simulink model "sat_model_delivery"  (R2023b)
settings: Solver=ode5  StartTime=0.0  StopTime=2*T  RelTol=1e-3
undefined symbols (not defined in the file): a, alpha1, alpha12, alpha2, alpha22, alpha3, bias_earth, bias_mag, bias_sun, DiscIntNeverNeededParam, e, flag_h, FOV_earth, freq_acds, freq_act, freq_earth, freq_mag, freq_sun, gh, I_ext, I_retr, I_wheel, Iinv_ext, Iinv_retr, jb, k_gain, magnitude, max_dip, max_hdot, mu, n, noise_sd_mag, omega0, omegaE, rs, s0, s_h, s_m, s_s, tol, v_h, v_m, v_s, w_sat
libraries: simulink x16, vrlib x10, matrix_library x7, cstextras x4, cstblocks x1, simulink_extras x1
(part 1 of 3)
settings Model: Creator=danie  LastModifiedBy=danie

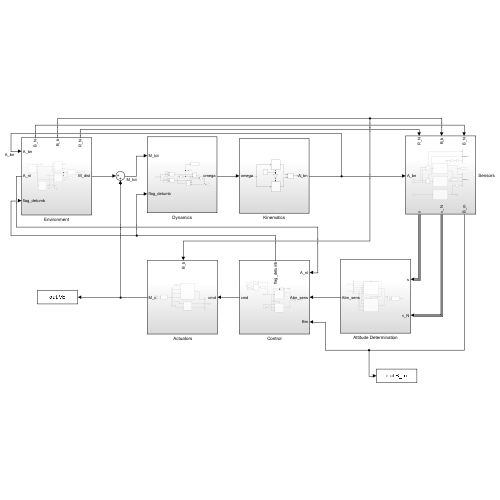
[thumbnail: Simulink's stored preview of the top-level diagram]
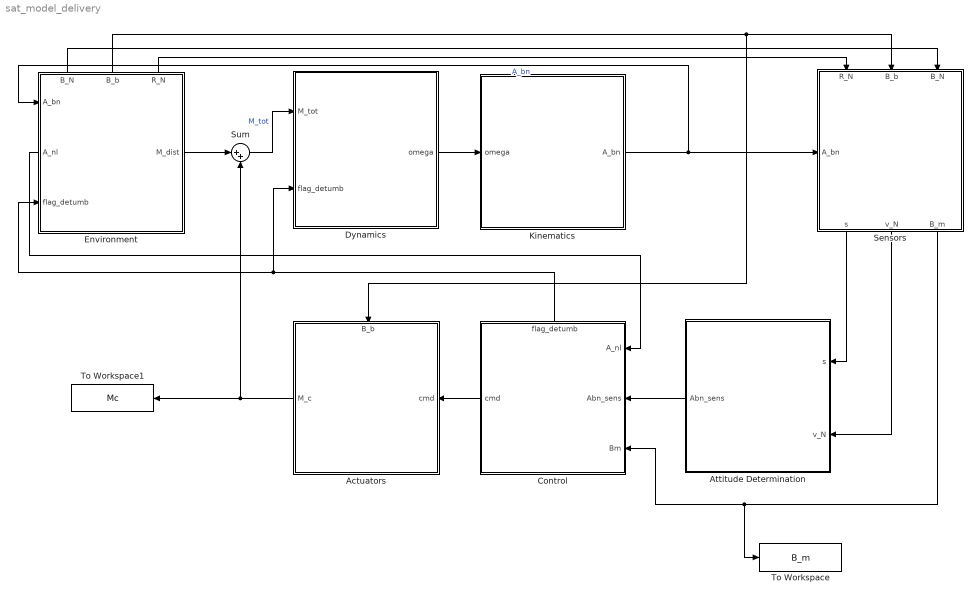
== system sat_model_delivery ==
  " Actuators" : Subsystem
      settings: PortSchema="{\"entries\":[{\"content\":{\"sides\":[{\"content\":{\"connectorIds\":[\"In1\"]},\"type\":\"ConnectorPlacement.EquallySpacedRectSide\",\"uuid\":\"5d6e642f-1157-4b0e-aa08-9ddf4ff16df7\"},{\"content\":{\"connectorIds\":[\"Out1\"],\"side\":\"RIGHT\"},\"type\":\"ConnectorPlacement.EquallySpacedRectSide\",\"uuid\":\"5847b5a1-e838-48cc-aba7-537ea27379c6\"},{\"content\":{\"connectorIds\":[\"In2\"],\"side\":\"TOP\"},\"type\":\"ConnectorPlacement.EquallySpacedRectSide\",\"uuid\":\"a1f0acea-f413-4d04-85a3-ab4e053335d5\"}]},\"type\":\"ConnectorPlacement.EquallySpacedConnector\",\"uuid\":\"33dffe5d-89c5-4628-a461-5573ab7b5256\"}],\"packageUris\":[\"http://schema.mathworks.com/mf0/Connector/R2020b\"],\"version\":\"1.0\"}"
  Attitude Determination : Subsystem
      settings: PortSchema="{\"entries\":[{\"content\":{\"sides\":[{\"content\":{\"connectorIds\":[\"Out1\"]},\"type\":\"ConnectorPlacement.EquallySpacedRectSide\",\"uuid\":\"730966cf-d0d7-44a0-92f0-b5324480e7cc\"},{\"content\":{\"connectorIds\":[\"In1\",\"In2\"],\"side\":\"RIGHT\"},\"type\":\"ConnectorPlacement.EquallySpacedRectSide\",\"uuid\":\"c83e6b57-46fe-4a45-9824-d3495e15bf6a\"},{\"content\":{\"side\":\"TOP\"},\"type\":\"ConnectorPlacement.EquallySpacedRectSide\",\"uuid\":\"4938c298-c2b3-45b7-bcb0-70b8132dabc6\"},{\"content\":{\"side\":\"BOTTOM\"},\"type\":\"ConnectorPlacement.EquallySpacedRectSide\",\"uuid\":\"6d6a244e-80db-423b-a0a5-9a5face48fcb\"}]},\"type\":\"ConnectorPlacement.EquallySpacedConnector\",\"uuid\":\"7eb6767d-3ff0-4577-86c9-ebc5e763f220\"}],\"packageUris\":[\"http://schema.mathworks.com/mf0/Connector/R2020b\"],\"version\":\"1.0\"}"
  Control : Subsystem
      settings: PortSchema="{\"entries\":[{\"content\":{\"sides\":[{\"content\":{\"connectorIds\":[\"In1\",\"In2\",\"In3\"]},\"type\":\"ConnectorPlacement.EquallySpacedRectSide\",\"uuid\":\"479db2a9-02dc-44e2-91e0-a22764ce85e5\"},{\"content\":{\"connectorIds\":[\"Out1\"],\"side\":\"RIGHT\"},\"type\":\"ConnectorPlacement.EquallySpacedRectSide\",\"uuid\":\"f4f8a6e1-932f-455d-9102-afbfd34f7a90\"},{\"content\":{\"connectorIds\":[\"Out2\"],\"side\":\"TOP\"},\"type\":\"ConnectorPlacement.EquallySpacedRectSide\",\"uuid\":\"6b9117e9-1db7-436f-b480-50cd5021b49c\"}]},\"type\":\"ConnectorPlacement.EquallySpacedConnector\",\"uuid\":\"5cd0260c-2101-4e31-9539-e0e89bfc4be8\"}],\"packageUris\":[\"http://schema.mathworks.com/mf0/Connector/R2020b\"],\"version\":\"1.0\"}"
  Dynamics : Subsystem
  Environment : Subsystem
      settings: PortSchema="{\"entries\":[{\"content\":{\"sides\":[{\"content\":{\"connectorIds\":[\"In1\",\"Out5\",\"In2\"]},\"type\":\"ConnectorPlacement.EquallySpacedRectSide\",\"uuid\":\"cd547eb7-7be0-4e5b-836c-c366b6478044\"},{\"content\":{\"connectorIds\":[\"Out1\"],\"side\":\"RIGHT\"},\"type\":\"ConnectorPlacement.EquallySpacedRectSide\",\"uuid\":\"e1dc659a-5264-4743-a04f-d64598214c88\"},{\"content\":{\"connectorIds\":[\"Out2\",\"Out3\",\"Out4\"],\"side\":\"TOP\"},\"type\":\"ConnectorPlacement.EquallySpacedRectSide\",\"uuid\":\"7e012610-9217-4888-a063-1dd5014a7789\"}]},\"type\":\"ConnectorPlacement.EquallySpacedConnector\",\"uuid\":\"403067f0-c93a-4211-8718-9c9152968794\"}],\"packageUris\":[\"http://schema.mathworks.com/mf0/Connector/R2020b\"],\"version\":\"1.0\"}"
  Kinematics : Subsystem
  Sensors : Subsystem
      settings: PortSchema="{\"entries\":[{\"content\":{\"sides\":[{\"content\":{\"connectorIds\":[\"In1\"]},\"type\":\"ConnectorPlacement.EquallySpacedRectSide\",\"uuid\":\"89361889-f7de-4872-ae0d-1858deeb7249\"},{\"content\":{\"side\":\"RIGHT\"},\"type\":\"ConnectorPlacement.EquallySpacedRectSide\",\"uuid\":\"dfd6afc4-03b7-4a72-bde7-03d61914b85e\"},{\"content\":{\"connectorIds\":[\"In2\",\"In3\",\"In4\"],\"side\":\"TOP\"},\"type\":\"ConnectorPlacement.EquallySpacedRectSide\",\"uuid\":\"ce9e53bd-32cb-428b-aff5-bfd70ec52f8d\"},{\"content\":{\"connectorIds\":[\"Out1\",\"Out2\",\"Out3\"],\"side\":\"BOTTOM\"},\"type\":\"ConnectorPlacement.EquallySpacedRectSide\",\"uuid\":\"2ad17a34-6232-44a6-b54d-45b43e2b5f52\"}]},\"type\":\"ConnectorPlacement.EquallySpacedConnector\",\"uuid\":\"a62cbf6d-d04c-4cf6-ac53-e5ea1ee04b12\"}],\"packageUris\":[\"http://schema.mathworks.com/mf0/Connector/R2020b\"],\"version\":\"1.0\"}"
  Sum : Sum  Inputs=|++
  To Workspace : ToWorkspace  VariableName=B_m  SampleTime=-1
  To Workspace1 : ToWorkspace  VariableName=Mc  SampleTime=-1
  wires:
  " Actuators"/1(M_c) -> To Workspace1/1, Sum/2
  Control/2(flag_detumb) -> Environment/2(flag_detumb), Dynamics/2(flag_detumb)
  Environment/2(B_N) -> Sensors/4(B_N)
  Control/1(cmd) -> " Actuators"/1(cmd)
  Environment/1(M_dist) -> Sum/1
  Kinematics/1(A_bn) -> Sensors/1(A_bn), Environment/1(A_bn)  "A_bn"
  Environment/4(R_N) -> Sensors/2(R_N)
  Attitude Determination/1(Abn_sens) -> Control/2(Abn_sens)
  Environment/3(B_b) -> " Actuators"/2(B_b), Sensors/3(B_b)
  Sensors/3(B_m) -> To Workspace/1, Control/3(Bm)
  Environment/5(A_nl) -> Control/1(A_nl)
  Sensors/1(s) -> Attitude Determination/1(s)
  Sensors/2(v_N) -> Attitude Determination/2(v_N)
  Dynamics/1(omega) -> Kinematics/1(omega)
  Sum/1 -> Dynamics/1(M_tot)  "M_tot"

== system sat_model_delivery/ Actuators ==
  cmd : Inport
  B_b : Inport  Port=2
  Constant : Constant  Value=5
  Demux : Demux  Outputs=5
  Discrete Varying Lowpass : Subsystem  mask(Discrete Varying Lowpass){N=2, w0=0, Ts=1/30}
      mask prompts: N "Control:simulink:VaryingLowpassLabel1"; w0 "Control:simulink:VaryingLowpassLabel2"; Ts "Control:simulink:VaryingLowpassLabel3"
      mask help: Control:simulink:VaryingLowpass2
      mask init:
      | if N~=round(N)
      |    hCB = get_param(gcb,'handle');
      |    DAStudio.slerror('Control:simulink:InvalidOrder',hCB)
      | elseif w0*Ts>=pi
      |    hCB = get_param(gcb,'handle');
      |    DAStudio.slerror('Control:simulink:InvalidPrewarp',hCB)
      | end
      | SimStatus = get_param(bdroot,'SimulationStatus');
      | if any(strcmp(SimStatus,{'initializing','updating','stopped'}))
      |    controllib.internal.blocks.varying.varyingLP(gcb,N,Ts)
      | end
      settings: LibrarySourceBlock=cstblocks/Linear Parameter Varying/Discrete Varying Lowpass
      mask Help: eval('helpview(''control'',''VaryingLowpassDT'');')
      mask DialogControl N Prompt: Filter order:
      mask DialogControl w0 Prompt: Pre-warping frequency w0 (rad/s):
      mask DialogControl Ts Prompt: Sample time Ts:
      mask Display:
      | image('lowpass_dt.png',[0.1 0 0.8 1]);
      | port_label('input', 2, 'freq');
  Magnetorquers : Subsystem
  Reaction wheels : Subsystem
  Sum : Sum  Inputs=+++
  M_c : Outport
  wires:
  Sum/1 -> M_c/1
  Constant/1 -> Discrete Varying Lowpass/2(frequency)
  Discrete Varying Lowpass/1(y) -> Demux/1
  cmd/1 -> Discrete Varying Lowpass/1(u)
  Demux/1 -> Magnetorquers/2(Dx)  "Dx"
  Demux/2 -> Magnetorquers/3(Dy)  "Dy"
  B_b/1 -> Magnetorquers/1(B_b)
  Demux/3 -> Magnetorquers/4(Dz)  "Dz"
  Magnetorquers/1(M_mag) -> Sum/1
  Demux/4 -> Reaction wheels/1(-h_dot_x)  "-h_dot_x"
  Demux/5 -> Reaction wheels/2(-h_dot_y)  "-h_dot_y"
  Reaction wheels/1(M_wheel_x) -> Sum/2
  Reaction wheels/2(M_wheel_y) -> Sum/3

== system sat_model_delivery/Attitude Determination ==
  s : Inport
  v_N : Inport  Port=2
  Bus Selector : BusSelector  OutputSignals=flag_h,s_h,s_s,s_m
  Bus Selector1 : BusSelector  OutputSignals=v_h,v_s,v_m
  Constant : Constant  Value=0.5
  Discrete Varying Lowpass : cstblocks/Linear Parameter Varying/Discrete Varying Lowpass  N=2  w0=0  Ts=1/freq_acds
  Merge : Merge
  NOT : Logic  Operator=NOT  IconShape=distinctive  AllPortsSameDT=off  OutDataTypeStr=boolean
  Three Sensors : Subsystem  TreatAsAtomicUnit=on
  Two Sensors : Subsystem  TreatAsAtomicUnit=on
  Abn_sens : Outport
  wires:
  Bus Selector/1 -> Three Sensors/Enable, NOT/1  "<flag_h>"
  NOT/1 -> Two Sensors/Enable
  Three Sensors/1(Abn_sens) -> Merge/1
  Two Sensors/1(A_bn_sens) -> Merge/2
  s/1 -> Bus Selector/1
  Bus Selector/2 -> Three Sensors/1(s1)  "<s_h>"
  Bus Selector/3 -> Two Sensors/1(s1), Three Sensors/2(s2)  "<s_s>"
  Bus Selector/4 -> Two Sensors/2(s2), Three Sensors/3(s3)  "<s_m>"
  v_N/1 -> Bus Selector1/1
  Bus Selector1/1 -> Three Sensors/4(v1)  "<v_h>"
  Bus Selector1/2 -> Two Sensors/3(v1), Three Sensors/5(v2)  "<v_s>"
  Bus Selector1/3 -> Two Sensors/4(v2), Three Sensors/6(v3)  "<v_m>"
  Merge/1 -> Discrete Varying Lowpass/1
  Discrete Varying Lowpass/1 -> Abn_sens/1
  Constant/1 -> Discrete Varying Lowpass/2

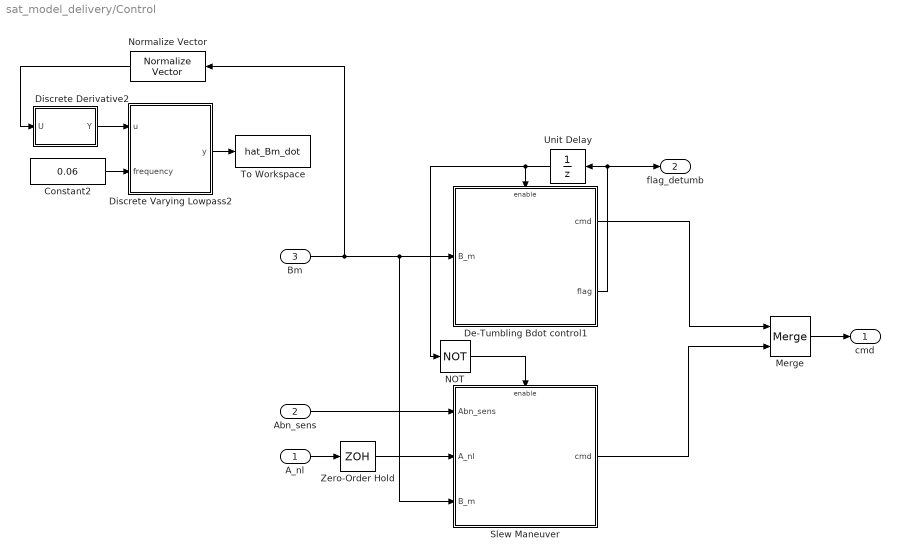
== system sat_model_delivery/Control ==
  A_nl : Inport
  Abn_sens : Inport  Port=2
  Bm : Inport  Port=3
  Constant2 : Constant  Value=0.06  SampleTime=1/freq_mag
  De-Tumbling Bdot control1 : Subsystem
  Discrete Derivative2 : Subsystem  mask(Discrete Derivative){gainval=1.0, ICPrevScaledInput=0, InputProcessing=Elements as channels (sample based), OutMin=[], OutMax=[], OutDataTypeStr=Inherit: Inherit via internal rule, OutputDataTypeScalingMode=Inherit via internal rule, OutDataType=fixdt(1, 16), OutScaling=2^-10, LockScale=off, RndMeth=Floor, DoSatur=off}
      mask prompts: gainval "Simulink:masks:GainValue_MP"; ICPrevScaledInput "Simulink:masks:InitialConditionForPreviousWeightedInputKuTs_MP"; InputProcessing "Simulink:masks:InputProcessing_MP"; OutMin "Simulink:masks:OutputMinimum_MP"; OutMax "Simulink:masks:OutputMaximum_MP"; OutDataTypeStr "Simulink:masks:OutputDataType_MP"; OutputDataTypeScalingMode "Simulink:masks:OutputDataTypeMode_MP"; OutDataType "Simulink:masks:OutputDataTypeegFixdt116Fixdtsingle_MP"; OutScaling "Simulink:masks:OutputScalingSlopeEg29OrSlopeBias_MP"; LockScale "Simulink:masks:LockOutputDataTypeAgainstFxpTools_MP"; RndMeth "Simulink:masks:IntegerRoundingMode_MP"; DoSatur "Simulink:masks:SaturateToMaxOrMinWhenOverflowsOccur_MP"
      mask help: Simulink:masks:DiscreteDerivative_MD
      mask init:
      | blkH = gcbh;
      | blkName = getfullname(blkH);
      | 
      | if (gainval == 0.0)
      |     %avoid divide by zero warning
      |     inverseGainval = inf;
      | else
      |     inverseGainval = 1.0/double(gainval);
      | end
      | 
      | if isequal(OutDataTypeStr, 'Inherit: Inherit via internal rule')
      |     diffDT   = 'Inherit: Inherit via back propagation';
      |     tsampDT  = 'Inherit: Inherit via internal rule';
      |     tsampImp = 'Offline Scaling Adjustment';
      | else    
      |     diffDT   = OutDataTypeStr;
      |     tsampDT  = 'Inherit: Inherit via back propagation';
      |     tsampImp = 'Online Calculations';
      | end
      | 
      | if ~strcmp(get_param(bdroot(blkH),'SimulationStatus'), 'running')
      |     set_param([blkName,'/Diff'], ...
      |               'RndMeth',RndMeth, ...
      | 	          'DoSatur',DoSatur);
      |     set_param([blkName,'/TSamp'], ...
      |               'OutDataTypeStr',tsampDT, ...
      |               'RndMeth',RndMeth, ...
      |               'DoSatur',DoSatur, ...
      |               'TsampMathImp',tsampImp);
      | end
      | 
      | set_param([blkName,'/UD'], ...
      | 	'InputProcessing',InputProcessing);
      settings: LibrarySourceBlock=simulink/Discrete/Discrete Derivative
      mask TypeOptions InputProcessing: Simulink:masks:ColumnsAsChannelsFrameBased | Simulink:masks:ElementsAsChannelsSampleBased
      mask Callback OutDataTypeStr: fixptdialog(gcbh)
      mask TypeOptions OutputDataTypeScalingMode: double | single | int8 | uint8 | int16 | uint16 | int32 | uint32 | Specify via dialog | Inherit via internal rule | Inherit via back propagation
      mask Callback OutputDataTypeScalingMode: fixptdialog(gcbh)
      mask Callback OutDataType: fixptdialog(gcbh)
      mask TypeOptions RndMeth: Simulink:masks:Ceiling | Simulink:masks:Convergent | Simulink:masks:Floor | Simulink:masks:Nearest | Simulink:masks:Round | Simulink:masks:Simplest | Simulink:masks:Zero
      mask Display: text(0.5, 0.5, 'K (z-1)', 'horizontalAlignment', 'center', 'verticalAlignment', 'bottom');text(0.5, 0.5, 'Ts z', 'horizontalAlignment', 'center', 'verticalAlignment', 'top');plot([0.3 0.7],[0.5 0.5]);
  Discrete Varying Lowpass2 : Subsystem  mask(Discrete Varying Lowpass){N=1, w0=0, Ts=1/freq_mag}
      mask prompts: N "Control:simulink:VaryingLowpassLabel1"; w0 "Control:simulink:VaryingLowpassLabel2"; Ts "Control:simulink:VaryingLowpassLabel3"
      mask help: Control:simulink:VaryingLowpass2
      mask init: same as sat_model_delivery/ Actuators/Discrete Varying Lowpass
      settings: LibrarySourceBlock=cstblocks/Linear Parameter Varying/Discrete Varying Lowpass
      mask Help: eval('helpview(''control'',''VaryingLowpassDT'');')
      mask DialogControl N Prompt: Filter order:
      mask DialogControl w0 Prompt: Pre-warping frequency w0 (rad/s):
      mask DialogControl Ts Prompt: Sample time Ts:
      mask Display:
      | image('lowpass_dt.png',[0.1 0 0.8 1]);
      | port_label('input', 2, 'freq');
  Merge : Merge
  NOT : Logic  Operator=NOT  IconShape=distinctive  AllPortsSameDT=off  OutDataTypeStr=boolean
  Normalize Vector : vrlib/Utilities/Normalize Vector  maxzero=0
  Slew Maneuver : Subsystem
  To Workspace : ToWorkspace  VariableName=hat_Bm_dot  SampleTime=-1
  Unit Delay : UnitDelay  InitialCondition=1  SampleTime=-1  HasFrameUpgradeWarning=on
  Zero-Order Hold : ZeroOrderHold  SampleTime=1/freq_acds
  cmd : Outport
  flag_detumb : Outport  Port=2
  wires:
  Unit Delay/1 -> NOT/1, De-Tumbling Bdot control1/Enable
  De-Tumbling Bdot control1/2(flag) -> flag_detumb/1, Unit Delay/1
  Bm/1 -> Normalize Vector/1, Slew Maneuver/3(B_m), De-Tumbling Bdot control1/1(B_m)
  Abn_sens/1 -> Slew Maneuver/1(Abn_sens)
  NOT/1 -> Slew Maneuver/Enable
  Slew Maneuver/1(cmd) -> Merge/2
  De-Tumbling Bdot control1/1(cmd) -> Merge/1
  A_nl/1 -> Zero-Order Hold/1
  Zero-Order Hold/1 -> Slew Maneuver/2(A_nl)
  Merge/1 -> cmd/1
  Constant2/1 -> Discrete Varying Lowpass2/2(frequency)
  Discrete Derivative2/1(Y) -> Discrete Varying Lowpass2/1(u)
  Discrete Varying Lowpass2/1(y) -> To Workspace/1
  Normalize Vector/1 -> Discrete Derivative2/1(U)

== system sat_model_delivery/Dynamics ==
  M_tot : Inport
  flag_detumb : Inport  Port=2
  Constant : Constant  Value=I_ext
  Constant1 : Constant  Value=Iinv_ext
  Constant2 : Constant  Value=I_retr
  Constant3 : Constant  Value=Iinv_retr
  Cross Product1 : matrix_library/Cross Product
  Integrator : Integrator  InitialCondition=omega0
  Product : Product  Multiplication=Matrix(*)
  Product1 : Product  Multiplication=Matrix(*)
  Sum : Sum  Inputs=++|
  Switch : Switch  Criteria=u2 ~= 0  SaturateOnIntegerOverflow=off  InputSameDT=off
  Switch1 : Switch  Criteria=u2 ~= 0  SaturateOnIntegerOverflow=off  InputSameDT=off
  To Workspace : ToWorkspace  VariableName=omega  SampleTime=-1
  omega : Outport
  wires:
  Product1/1 -> Integrator/1  "omega_dot"
  Integrator/1 -> omega/1, To Workspace/1, Cross Product1/2, Product/2  "omega"
  Product/1 -> Cross Product1/1
  Cross Product1/1 -> Sum/1
  Sum/1 -> Product1/2
  M_tot/1 -> Sum/2
  flag_detumb/1 -> Switch/2, Switch1/2
  Constant2/1 -> Switch/1
  Constant/1 -> Switch/3
  Constant1/1 -> Switch1/3
  Constant3/1 -> Switch1/1
  Switch/1 -> Product/1
  Switch1/1 -> Product1/1

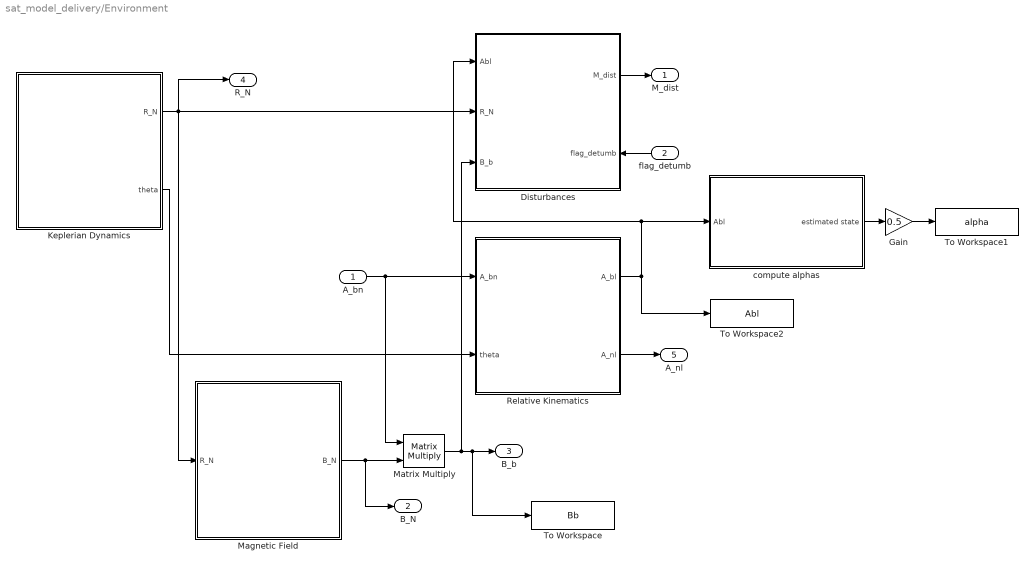
== system sat_model_delivery/Environment ==
  A_bn : Inport
  flag_detumb : Inport  Port=2
  Disturbances : Subsystem
      settings: PortSchema="{\"entries\":[{\"content\":{\"sides\":[{\"content\":{\"connectorIds\":[\"In1\",\"In2\",\"In3\"]},\"type\":\"ConnectorPlacement.EquallySpacedRectSide\",\"uuid\":\"a54a8b75-5c45-4c9d-a840-4100710c8f73\"},{\"content\":{\"connectorIds\":[\"Out1\",\"In4\"],\"side\":\"RIGHT\"},\"type\":\"ConnectorPlacement.EquallySpacedRectSide\",\"uuid\":\"db0184ce-e0b6-40fa-9e41-5dcbbcff6eec\"},{\"content\":{\"side\":\"TOP\"},\"type\":\"ConnectorPlacement.EquallySpacedRectSide\",\"uuid\":\"aace9336-137f-4243-910d-085c66e24849\"}]},\"type\":\"ConnectorPlacement.EquallySpacedConnector\",\"uuid\":\"c00bf988-d11b-409b-9760-08537e3b8bbd\"}],\"packageUris\":[\"http://schema.mathworks.com/mf0/Connector/R2020b\"],\"version\":\"1.0\"}"
  Gain : Gain  Gain=0.5
  Keplerian Dynamics : Subsystem
  Magnetic Field : Subsystem
  Matrix Multiply : Product  Multiplication=Matrix(*)
  Relative Kinematics : Subsystem
  To Workspace : ToWorkspace  VariableName=Bb  SampleTime=-1
  To Workspace1 : ToWorkspace  VariableName=alpha  SampleTime=-1
  To Workspace2 : ToWorkspace  VariableName=Abl  SampleTime=-1
  compute alphas : Subsystem
  M_dist : Outport
  B_N : Outport  Port=2
  B_b : Outport  Port=3
  R_N : Outport  Port=4
  A_nl : Outport  Port=5
  wires:
  Keplerian Dynamics/1(R_N) -> R_N/1, Disturbances/2(R_N), Magnetic Field/1(R_N)
  Disturbances/1(M_dist) -> M_dist/1
  Keplerian Dynamics/2(theta) -> Relative Kinematics/2(theta)
  A_bn/1 -> Relative Kinematics/1(A_bn), Matrix Multiply/1
  Relative Kinematics/1(A_bl) -> To Workspace2/1, compute alphas/1(Abl), Disturbances/1(Abl)
  Magnetic Field/1(B_N) -> B_N/1, Matrix Multiply/2
  Matrix Multiply/1 -> To Workspace/1, B_b/1, Disturbances/3(B_b)
  Relative Kinematics/2(A_nl) -> A_nl/1
  flag_detumb/1 -> Disturbances/4(flag_detumb)
  compute alphas/1(estimated state) -> Gain/1
  Gain/1 -> To Workspace1/1

== system sat_model_delivery/Kinematics ==
  omega : Inport
  Kinematics 312 : Subsystem
  Kinematics 313 : Subsystem
  Merge : Merge
  NOT : Logic  Operator=NOT  IconShape=distinctive  AllPortsSameDT=off  OutDataTypeStr=boolean
  System switcher : Subsystem
  A_bn : Outport
  wires:
  NOT/1 -> Kinematics 313/Enable
  omega/1 -> Kinematics 312/1(w), Kinematics 313/1(w)
  System switcher/1(flag) -> Kinematics 312/Enable, NOT/1
  Kinematics 313/1(A) -> Merge/2
  Merge/1 -> A_bn/1
  Kinematics 312/1(A) -> Merge/1

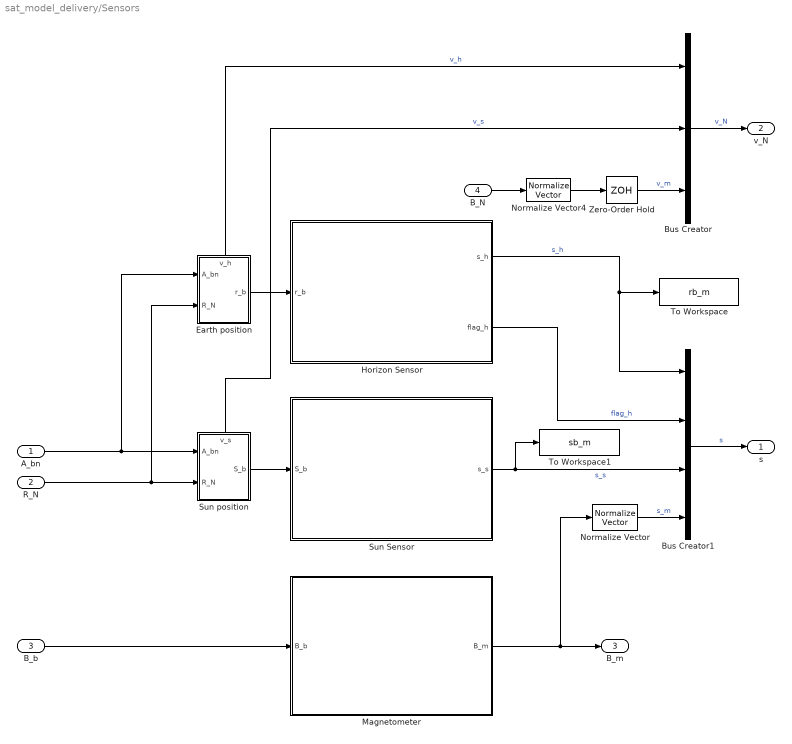
== system sat_model_delivery/Sensors ==
  A_bn : Inport
  R_N : Inport  Port=2
  B_b : Inport  Port=3
  B_N : Inport  Port=4
  Bus Creator : BusCreator  Inputs=v_h,v_s,v_m
  Bus Creator1 : BusCreator  Inputs=s_h,flag_h,s_s,s_m
  Earth position : Subsystem
      settings: PortSchema="{\"entries\":[{\"content\":{\"sides\":[{\"content\":{\"connectorIds\":[\"In1\",\"In2\"]},\"type\":\"ConnectorPlacement.EquallySpacedRectSide\",\"uuid\":\"035c2cbe-782b-4a42-a6ee-6bd5e444eb90\"},{\"content\":{\"connectorIds\":[\"Out1\"],\"side\":\"RIGHT\"},\"type\":\"ConnectorPlacement.EquallySpacedRectSide\",\"uuid\":\"508f84b9-68d8-43ca-a052-308802da088c\"},{\"content\":{\"connectorIds\":[\"Out2\"],\"side\":\"TOP\"},\"type\":\"ConnectorPlacement.EquallySpacedRectSide\",\"uuid\":\"f659f755-28ee-4a7b-8f7a-331900bd0b68\"}]},\"type\":\"ConnectorPlacement.EquallySpacedConnector\",\"uuid\":\"dca93633-1f86-4f52-a614-75741afaac51\"}],\"packageUris\":[\"http://schema.mathworks.com/mf0/Connector/R2020b\"],\"version\":\"1.0\"}"
  Horizon Sensor : Subsystem
  Magnetometer : Subsystem
  Normalize Vector : vrlib/Utilities/Normalize Vector  maxzero=0
  Normalize Vector4 : vrlib/Utilities/Normalize Vector  maxzero=0
  Sun Sensor : Subsystem
  Sun position : Subsystem
      settings: PortSchema="{\"entries\":[{\"content\":{\"sides\":[{\"content\":{\"connectorIds\":[\"In1\",\"In2\"]},\"type\":\"ConnectorPlacement.EquallySpacedRectSide\",\"uuid\":\"035c2cbe-782b-4a42-a6ee-6bd5e444eb90\"},{\"content\":{\"connectorIds\":[\"Out1\"],\"side\":\"RIGHT\"},\"type\":\"ConnectorPlacement.EquallySpacedRectSide\",\"uuid\":\"508f84b9-68d8-43ca-a052-308802da088c\"},{\"content\":{\"connectorIds\":[\"Out2\"],\"side\":\"TOP\"},\"type\":\"ConnectorPlacement.EquallySpacedRectSide\",\"uuid\":\"f659f755-28ee-4a7b-8f7a-331900bd0b68\"},{\"content\":{\"side\":\"BOTTOM\"},\"type\":\"ConnectorPlacement.EquallySpacedRectSide\",\"uuid\":\"e8854be4-8231-4a4d-8c90-98d0dafc83b2\"}]},\"type\":\"ConnectorPlacement.EquallySpacedConnector\",\"uuid\":\"dca93633-1f86-4f52-a614-75741afaac51\"}],\"packageUris\":[\"http://schema.mathworks.com/mf0/Connector/R2020b\"],\"version\":\"1.0\"}"
  To Workspace : ToWorkspace  VariableName=rb_m  SampleTime=-1
  To Workspace1 : ToWorkspace  VariableName=sb_m  SampleTime=-1
  Zero-Order Hold : ZeroOrderHold  SampleTime=1/freq_acds
  s : Outport
  v_N : Outport  Port=2
  B_m : Outport  Port=3
  wires:
  B_b/1 -> Magnetometer/1(B_b)
  Sun position/1(S_b) -> Sun Sensor/1(S_b)
  R_N/1 -> Earth position/2(R_N), Sun position/2(R_N)
  A_bn/1 -> Earth position/1(A_bn), Sun position/1(A_bn)
  Earth position/1(r_b) -> Horizon Sensor/1(r_b)
  Normalize Vector4/1 -> Zero-Order Hold/1
  B_N/1 -> Normalize Vector4/1
  Earth position/2(v_h) -> Bus Creator/1  "v_h"
  Sun position/2(v_s) -> Bus Creator/2  "v_s"
  Bus Creator/1 -> v_N/1  "v_N"
  Bus Creator1/1 -> s/1  "s"
  Horizon Sensor/1(s_h) -> Bus Creator1/1, To Workspace/1  "s_h"
  Horizon Sensor/2(flag_h) -> Bus Creator1/2  "flag_h"
  Sun Sensor/1(s_s) -> To Workspace1/1, Bus Creator1/3  "s_s"
  Magnetometer/1("B_m ") -> B_m/1, Normalize Vector/1
  Zero-Order Hold/1 -> Bus Creator/3  "v_m"
  Normalize Vector/1 -> Bus Creator1/4  "s_m"

== system sat_model_delivery/ Actuators/Discrete Varying Lowpass ==
  u : Inport
  frequency : Inport  Port=2
  SOS1 : cstextras/DiscreteSecondOrderSection  VariantControl=order2  zeta=sin(1*pi/4)  Ts=Ts  w0=w0
  y : Outport  VectorParamsAs1DForOutWhenUnconnected=off
  wires:
  u/1 -> SOS1/1
  frequency/1 -> SOS1/2
  SOS1/1 -> y/1

== system sat_model_delivery/ Actuators/Magnetorquers ==
  B_b : Inport
  Dx : Inport  Port=2
  Dy : Inport  Port=3
  Dz : Inport  Port=4
  Band-Limited White Noise : simulink/Sources/Band-Limited White Noise  Cov=(1e-3*max_dip)^2/freq_act  Ts=1/freq_act  seed=[23341]
  Band-Limited White Noise1 : simulink/Sources/Band-Limited White Noise  Cov=(1e-3*max_dip)^2/freq_act  Ts=1/freq_act  seed=[23341]
  Band-Limited White Noise2 : simulink/Sources/Band-Limited White Noise  Cov=(1e-3*max_dip)^2/freq_act  Ts=1/freq_act  seed=[23341]
  Cross Product1 : matrix_library/Cross Product
  Rate Limiter1 : RateLimiter  RisingSlewLimit=100  FallingSlewLimit=-100
  Saturation : Saturate  UpperLimit=max_dip  LowerLimit=-max_dip
  Sum2 : Sum  Inputs=++|
  Vector Concatenate : Concatenate  NumInputs=3
  Vector Concatenate1 : Concatenate  NumInputs=3
  M_mag : Outport
  wires:
  B_b/1 -> Cross Product1/2
  Rate Limiter1/1 -> Saturation/1
  Dx/1 -> Vector Concatenate/1
  Cross Product1/1 -> M_mag/1
  Dz/1 -> Vector Concatenate/3
  Dy/1 -> Vector Concatenate/2
  Band-Limited White Noise/1 -> Vector Concatenate1/1
  Band-Limited White Noise1/1 -> Vector Concatenate1/2
  Band-Limited White Noise2/1 -> Vector Concatenate1/3
  Saturation/1 -> Sum2/2
  Sum2/1 -> Cross Product1/1
  Vector Concatenate/1 -> Rate Limiter1/1
  Vector Concatenate1/1 -> Sum2/1

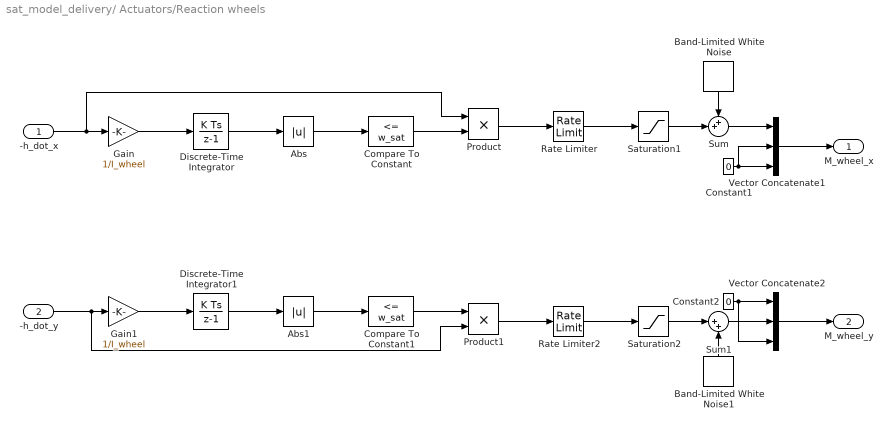
== system sat_model_delivery/ Actuators/Reaction wheels ==
  -h_dot_x : Inport
  -h_dot_y : Inport  Port=2
  Abs : Abs  SaturateOnIntegerOverflow=off
  Abs1 : Abs  SaturateOnIntegerOverflow=off
  Band-Limited White Noise : simulink/Sources/Band-Limited White Noise  Cov=(max_hdot*1e-5)^2/freq_act  Ts=1/freq_act  seed=[23341]
  Band-Limited White Noise1 : simulink/Sources/Band-Limited White Noise  Cov=(max_hdot*1e-5)^2/freq_act  Ts=1/freq_act  seed=[23341]
  Compare To Constant : simulink/Logic and Bit Operations/Compare To Constant  relop=<=  const=w_sat  OutDataTypeStr=boolean
  Compare To Constant1 : simulink/Logic and Bit Operations/Compare To Constant  relop=<=  const=w_sat  OutDataTypeStr=boolean
  Constant1 : Constant  Value=0
  Constant2 : Constant  Value=0
  Discrete-Time Integrator : DiscreteIntegrator  SampleTime=-1  ICPrevOutput=DiscIntNeverNeededParam  ICPrevScaledInput=DiscIntNeverNeededParam
  Discrete-Time Integrator1 : DiscreteIntegrator  SampleTime=-1  ICPrevOutput=DiscIntNeverNeededParam  ICPrevScaledInput=DiscIntNeverNeededParam
  Gain : Gain  Gain=1/I_wheel
  Gain1 : Gain  Gain=1/I_wheel
  Product : Product
  Product1 : Product
  Rate Limiter : RateLimiter
  Rate Limiter2 : RateLimiter
  Saturation1 : Saturate  UpperLimit=max_hdot  LowerLimit=-max_hdot
  Saturation2 : Saturate  UpperLimit=max_hdot  LowerLimit=-max_hdot
  Sum : Sum  Inputs=++|
  Sum1 : Sum  Inputs=|++
  Vector Concatenate1 : Concatenate  NumInputs=3
  Vector Concatenate2 : Concatenate  NumInputs=3
  M_wheel_x : Outport
  M_wheel_y : Outport  Port=2
  wires:
  Constant1/1 -> Vector Concatenate1/3, Vector Concatenate1/2
  Rate Limiter/1 -> Saturation1/1
  Rate Limiter2/1 -> Saturation2/1
  -h_dot_x/1 -> Gain/1, Product/1
  Vector Concatenate1/1 -> M_wheel_x/1
  Vector Concatenate2/1 -> M_wheel_y/1
  -h_dot_y/1 -> Gain1/1, Product1/2
  Gain/1 -> Discrete-Time Integrator/1
  Gain1/1 -> Discrete-Time Integrator1/1
  Discrete-Time Integrator1/1 -> Abs1/1
  Compare To Constant/1 -> Product/2
  Product/1 -> Rate Limiter/1
  Compare To Constant1/1 -> Product1/1
  Product1/1 -> Rate Limiter2/1
  Constant2/1 -> Vector Concatenate2/3, Vector Concatenate2/1
  Discrete-Time Integrator/1 -> Abs/1
  Abs/1 -> Compare To Constant/1
  Abs1/1 -> Compare To Constant1/1
  Saturation1/1 -> Sum/2
  Sum/1 -> Vector Concatenate1/1
  Saturation2/1 -> Sum1/1
  Sum1/1 -> Vector Concatenate2/2
  Band-Limited White Noise/1 -> Sum/1
  Band-Limited White Noise1/1 -> Sum1/2

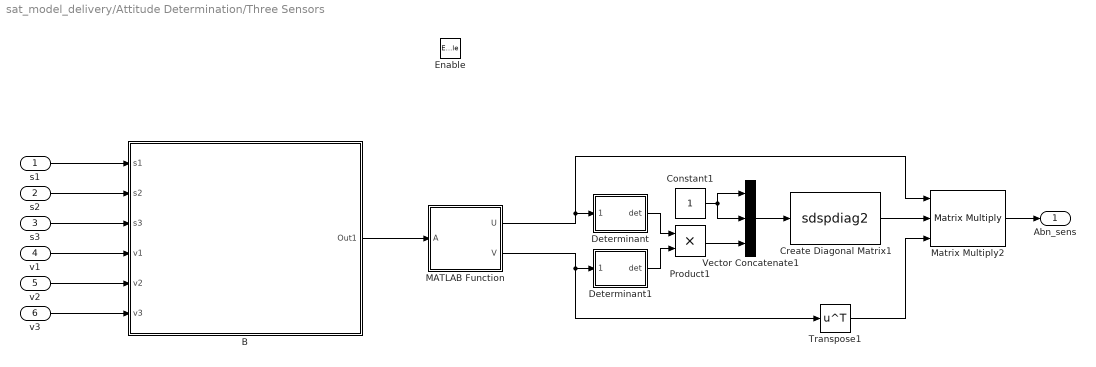
== system sat_model_delivery/Attitude Determination/Three Sensors ==
  s1 : Inport
  s2 : Inport  Port=2
  s3 : Inport  Port=3
  v1 : Inport  Port=4
  v2 : Inport  Port=5
  v3 : Inport  Port=6
  Enable : EnablePort
  B : Subsystem
  Constant1 : Constant
  Create Diagonal Matrix1 : S-Function  FunctionName=sdspdiag2  Parameters=mode  SFunctionDeploymentMode=off  EnableBusSupport=off  mask(Create Diagonal Matrix){}
      mask help: Simulink:masks:CreateDiagonalMatrix_MD
      mask init:
      | mode = 1;
      settings: LibrarySourceBlock=|
      | simulink/Matrix
      | Operations/Create Diagonal
      | Matrix
      mask Display:
      | x = [.58 .87 .87 .58 .58 NaN 0.45 0.12 NaN 0.525 0.525 0.475 0.475 0.525 0.525 0.565 0.525 ];
      | y = [ 0.2 0.2 0.8 0.8 0.2 NaN 0.2 0.8 NaN 0.435 0.475 0.475 0.525 0.525 0.565 0.5 0.435 ];
      | plot(x,y);
      | port_label('input',1,'D');
      | port_label('output',1,'A');
  Determinant : Subsystem
      settings: LibrarySourceBlock=|
      | aerolibutil/Determinant of
      | 3x3 Matrix
  Determinant1 : Subsystem
      settings: LibrarySourceBlock=|
      | aerolibutil/Determinant of
      | 3x3 Matrix
  MATLAB Function : MATLAB Function  TreatAsAtomicUnit=on
  Matrix Multiply2 : Product  Inputs=3  Multiplication=Matrix(*)
  Product1 : Product
  Transpose1 : Math  Operator=transpose
  Vector Concatenate1 : Concatenate  NumInputs=3
  Abn_sens : Outport
  wires:
  MATLAB Function/2(V) -> Determinant1/1(Matrix), Transpose1/1
  MATLAB Function/1(U) -> Determinant/1(Matrix), Matrix Multiply2/1
  Vector Concatenate1/1 -> Create Diagonal Matrix1/1
  Transpose1/1 -> Matrix Multiply2/3
  Determinant1/1(det) -> Product1/2
  Product1/1 -> Vector Concatenate1/3
  Create Diagonal Matrix1/1 -> Matrix Multiply2/2
  Constant1/1 -> Vector Concatenate1/2, Vector Concatenate1/1
  Determinant/1(det) -> Product1/1
  B/1(Out1) -> MATLAB Function/1(A)
  s1/1 -> B/1(s1)
  s2/1 -> B/2(s2)
  s3/1 -> B/3(s3)
  v1/1 -> B/4(v1)
  v2/1 -> B/5(v2)
  v3/1 -> B/6(v3)
  Matrix Multiply2/1 -> Abn_sens/1

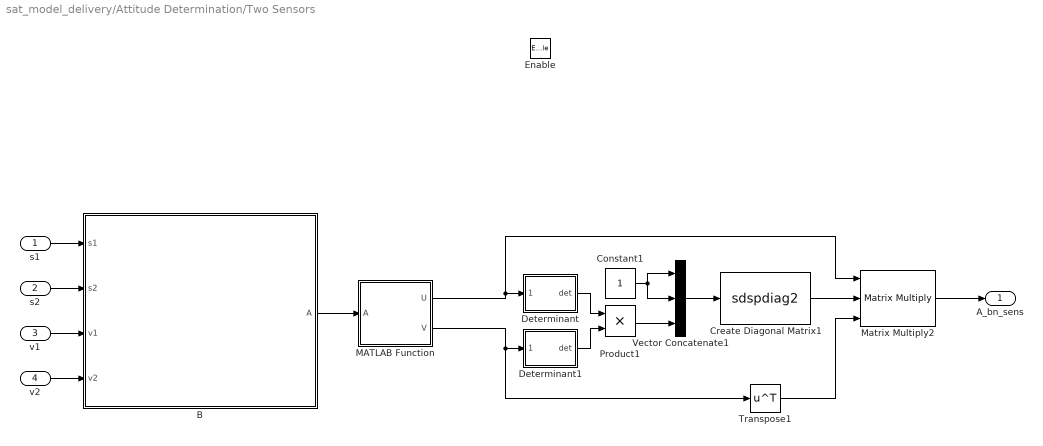
== system sat_model_delivery/Attitude Determination/Two Sensors ==
  s1 : Inport
  s2 : Inport  Port=2
  v1 : Inport  Port=3
  v2 : Inport  Port=4
  Enable : EnablePort
  B : Subsystem
  Constant1 : Constant
  Create Diagonal Matrix1 : S-Function  FunctionName=sdspdiag2  Parameters=mode  SFunctionDeploymentMode=off  EnableBusSupport=off  mask(Create Diagonal Matrix){}
      mask help: Simulink:masks:CreateDiagonalMatrix_MD
      mask init:
      | mode = 1;
      settings: LibrarySourceBlock=|
      | simulink/Matrix
      | Operations/Create Diagonal
      | Matrix
      mask Display:
      | x = [.58 .87 .87 .58 .58 NaN 0.45 0.12 NaN 0.525 0.525 0.475 0.475 0.525 0.525 0.565 0.525 ];
      | y = [ 0.2 0.2 0.8 0.8 0.2 NaN 0.2 0.8 NaN 0.435 0.475 0.475 0.525 0.525 0.565 0.5 0.435 ];
      | plot(x,y);
      | port_label('input',1,'D');
      | port_label('output',1,'A');
  Determinant : Subsystem
      settings: LibrarySourceBlock=|
      | aerolibutil/Determinant of
      | 3x3 Matrix
  Determinant1 : Subsystem
      settings: LibrarySourceBlock=|
      | aerolibutil/Determinant of
      | 3x3 Matrix
  MATLAB Function : MATLAB Function  TreatAsAtomicUnit=on
  Matrix Multiply2 : Product  Inputs=3  Multiplication=Matrix(*)
  Product1 : Product
  Transpose1 : Math  Operator=transpose
  Vector Concatenate1 : Concatenate  NumInputs=3
  A_bn_sens : Outport
  wires:
  v2/1 -> B/4(v2)
  v1/1 -> B/3(v1)
  s2/1 -> B/2(s2)
  s1/1 -> B/1(s1)
  Create Diagonal Matrix1/1 -> Matrix Multiply2/2
  Transpose1/1 -> Matrix Multiply2/3
  Product1/1 -> Vector Concatenate1/3
  MATLAB Function/1(U) -> Determinant/1(Matrix), Matrix Multiply2/1
  Constant1/1 -> Vector Concatenate1/2, Vector Concatenate1/1
  Determinant1/1(det) -> Product1/2
  MATLAB Function/2(V) -> Determinant1/1(Matrix), Transpose1/1
  Determinant/1(det) -> Product1/1
  Vector Concatenate1/1 -> Create Diagonal Matrix1/1
  Matrix Multiply2/1 -> A_bn_sens/1
  B/1(A) -> MATLAB Function/1(A)

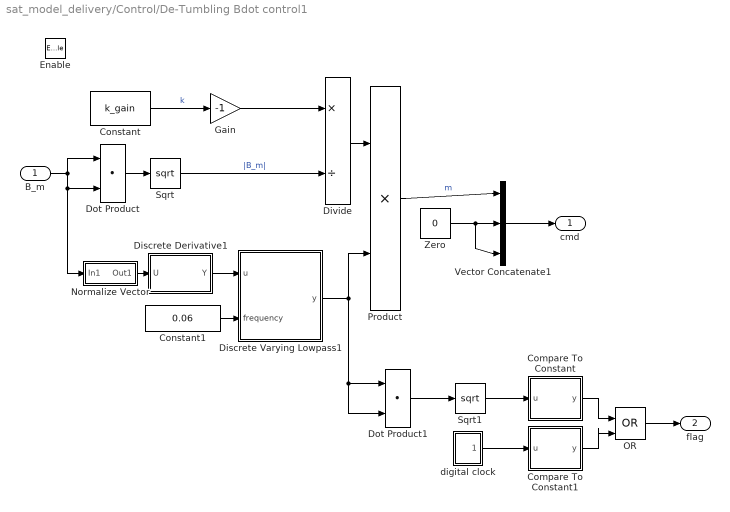
== system sat_model_delivery/Control/De-Tumbling Bdot control1 ==
  B_m : Inport
  Enable : EnablePort
  Compare To Constant : Subsystem  mask(Compare To Constant){relop=>=, const=0.003, OutDataTypeStr=boolean, ZeroCross=on}
      mask prompts: relop "Simulink:masks:Operator_MP"; const "Simulink:masks:ConstantValue_MP"; OutDataTypeStr "Simulink:masks:OutputDataType_MP"; ZeroCross "Simulink:masks:EnableZerocrossingDetection_MP"
      mask help: Simulink:masks:CompareToConstant_MD
      mask init:
      | blkName = gcb;
      | 
      | if strcmp(get_param(gcbh,'OutDataTypeStr'),'boolean')
      | 	setValue = 'boolean';
      | else
      | 	setValue = 'fixdt(0, 8, 0)';
      | end
      | 
      | set_param([blkName,'/Compare'],'relop',relop, ...
      | 	'OutDataTypeStr', setValue, 'ZeroCross', ZeroCross);
      | 
      | str = [relop,' C']; %default
      | 
      | const_str = get_param(blkName, 'const');
      | const_val = str2num(const_str);
      | 
      | if isempty(const_val) %#ok<ST2NM>
      |     %Expression/Variable
      |     str = [relop, ' ', strtrim(const_str)];
      | else
      |     if length(const_val) == 1 
      |         if Simulink.data.isSupportedEnumClass(class(const_val))
      |             % Special Handling for Enumerations
      |             if Simulink.data.getEnumTypeInfo(class(const_val), 'AddClassNameToEnumNames')
      |                 str = [relop, ' ', strtrim(const_str)];
      |             else
      |                 str = [relop, ' ', char(const_val)];
      |             end
      |         elseif(isfloat(const_val) || isinteger(const_val) || islogical(const_val)) 
      |                 str = [relop, ' ', num2str(const_val)];
      |         end
      |     end
      | end
      settings: LibrarySourceBlock=|
      | simulink/Logic and Bit
      | Operations/Compare
      | To Constant
      mask TypeOptions relop: == | ~= | < | <= | >= | >
      mask TypeOptions OutDataTypeStr: Simulink:masks:uint8 | Simulink:masks:boolean
      mask Callback ZeroCross: sl('zeroCrossEnable', gcbh);
      mask Display: disp(str)
  Compare To Constant1 : Subsystem  mask(Compare To Constant){relop=<=, const=10, OutDataTypeStr=boolean, ZeroCross=on}
      mask prompts: relop "Simulink:masks:Operator_MP"; const "Simulink:masks:ConstantValue_MP"; OutDataTypeStr "Simulink:masks:OutputDataType_MP"; ZeroCross "Simulink:masks:EnableZerocrossingDetection_MP"
      mask help: Simulink:masks:CompareToConstant_MD
      mask init: same as sat_model_delivery/Control/De-Tumbling Bdot control1/Compare To Constant
      settings: LibrarySourceBlock=|
      | simulink/Logic and Bit
      | Operations/Compare
      | To Constant
      mask TypeOptions relop: == | ~= | < | <= | >= | >
      mask TypeOptions OutDataTypeStr: Simulink:masks:uint8 | Simulink:masks:boolean
      mask Callback ZeroCross: sl('zeroCrossEnable', gcbh);
      mask Display: disp(str)
  Constant : Constant  Value=k_gain
  Constant1 : Constant  Value=0.06  SampleTime=1/freq_mag
  Discrete Derivative1 : Subsystem  mask(Discrete Derivative){gainval=1.0, ICPrevScaledInput=0, InputProcessing=Elements as channels (sample based), OutMin=[], OutMax=[], OutDataTypeStr=Inherit: Inherit via internal rule, OutputDataTypeScalingMode=Inherit via internal rule, OutDataType=fixdt(1, 16), OutScaling=2^-10, LockScale=off, RndMeth=Floor, DoSatur=off}
      mask prompts: gainval "Simulink:masks:GainValue_MP"; ICPrevScaledInput "Simulink:masks:InitialConditionForPreviousWeightedInputKuTs_MP"; InputProcessing "Simulink:masks:InputProcessing_MP"; OutMin "Simulink:masks:OutputMinimum_MP"; OutMax "Simulink:masks:OutputMaximum_MP"; OutDataTypeStr "Simulink:masks:OutputDataType_MP"; OutputDataTypeScalingMode "Simulink:masks:OutputDataTypeMode_MP"; OutDataType "Simulink:masks:OutputDataTypeegFixdt116Fixdtsingle_MP"; OutScaling "Simulink:masks:OutputScalingSlopeEg29OrSlopeBias_MP"; LockScale "Simulink:masks:LockOutputDataTypeAgainstFxpTools_MP"; RndMeth "Simulink:masks:IntegerRoundingMode_MP"; DoSatur "Simulink:masks:SaturateToMaxOrMinWhenOverflowsOccur_MP"
      mask help: Simulink:masks:DiscreteDerivative_MD
      mask init: same as sat_model_delivery/Control/Discrete Derivative2
      settings: LibrarySourceBlock=simulink/Discrete/Discrete Derivative
      mask TypeOptions InputProcessing: Simulink:masks:ColumnsAsChannelsFrameBased | Simulink:masks:ElementsAsChannelsSampleBased
      mask Callback OutDataTypeStr: fixptdialog(gcbh)
      mask TypeOptions OutputDataTypeScalingMode: double | single | int8 | uint8 | int16 | uint16 | int32 | uint32 | Specify via dialog | Inherit via internal rule | Inherit via back propagation
      mask Callback OutputDataTypeScalingMode: fixptdialog(gcbh)
      mask Callback OutDataType: fixptdialog(gcbh)
      mask TypeOptions RndMeth: Simulink:masks:Ceiling | Simulink:masks:Convergent | Simulink:masks:Floor | Simulink:masks:Nearest | Simulink:masks:Round | Simulink:masks:Simplest | Simulink:masks:Zero
      mask Display: text(0.5, 0.5, 'K (z-1)', 'horizontalAlignment', 'center', 'verticalAlignment', 'bottom');text(0.5, 0.5, 'Ts z', 'horizontalAlignment', 'center', 'verticalAlignment', 'top');plot([0.3 0.7],[0.5 0.5]);
  Discrete Varying Lowpass1 : Subsystem  mask(Discrete Varying Lowpass){N=1, w0=0, Ts=1/freq_mag}
      mask prompts: N "Control:simulink:VaryingLowpassLabel1"; w0 "Control:simulink:VaryingLowpassLabel2"; Ts "Control:simulink:VaryingLowpassLabel3"
      mask help: Control:simulink:VaryingLowpass2
      mask init: same as sat_model_delivery/ Actuators/Discrete Varying Lowpass
      settings: LibrarySourceBlock=cstblocks/Linear Parameter Varying/Discrete Varying Lowpass
      mask Help: eval('helpview(''control'',''VaryingLowpassDT'');')
      mask DialogControl N Prompt: Filter order:
      mask DialogControl w0 Prompt: Pre-warping frequency w0 (rad/s):
      mask DialogControl Ts Prompt: Sample time Ts:
      mask Display:
      | image('lowpass_dt.png',[0.1 0 0.8 1]);
      | port_label('input', 2, 'freq');
  Divide : Product  Inputs=*/
  Dot Product : DotProduct  OutDataTypeStr=Inherit: Inherit via internal rule
  Dot Product1 : DotProduct  OutDataTypeStr=Inherit: Inherit via internal rule
  Gain : Gain  Gain=-1
  Normalize Vector : Subsystem  mask(Normalize Vector){maxzero=0}
      mask prompts: maxzero "Maximum modulus to treat vector as zero:"
      mask help:
      | Normalize a vector.
      | Output is the unit vector parallel to the input vector. Input can be vector of any size.
      | If the modulus of the input is lower or equal than specified, the output is set to zeros(size(u)).
      settings: LibrarySourceBlock=vrlib/Utilities/Normalize Vector
      mask Help: helpview(vrmfunc('FnHelpTopic'), 'vr_normalizevector');
      mask Display: disp('Normalize')
  OR : Logic  Operator=OR  IconShape=distinctive  AllPortsSameDT=off  OutDataTypeStr=boolean
  Product : Product
  Sqrt : Sqrt
  Sqrt1 : Sqrt
  Vector Concatenate1 : Concatenate  NumInputs=3
  Zero : Constant  Value=0  OutDataTypeStr=Inherit: Inherit via back propagation
  digital clock : Subsystem
  cmd : Outport
  flag : Outport  Port=2
  wires:
  Dot Product/1 -> Sqrt/1
  Constant/1 -> Gain/1  "k"
  Divide/1 -> Product/1
  Product/1 -> Vector Concatenate1/1  "m"
  Sqrt/1 -> Divide/2  "|B_m|"
  Gain/1 -> Divide/1
  Normalize Vector/1(Out1) -> Discrete Derivative1/1(U)
  B_m/1 -> Dot Product/2, Normalize Vector/1(In1), Dot Product/1
  Discrete Derivative1/1(Y) -> Discrete Varying Lowpass1/1(u)
  Sqrt1/1 -> Compare To Constant/1(u)
  Dot Product1/1 -> Sqrt1/1
  OR/1 -> flag/1
  Compare To Constant/1(y) -> OR/1
  Compare To Constant1/1(y) -> OR/2
  Constant1/1 -> Discrete Varying Lowpass1/2(frequency)
  Discrete Varying Lowpass1/1(y) -> Dot Product1/2, Dot Product1/1, Product/2
  Vector Concatenate1/1 -> cmd/1
  Zero/1 -> Vector Concatenate1/3, Vector Concatenate1/2
  digital clock/1(Out1) -> Compare To Constant1/1(u)

== system sat_model_delivery/Control/Discrete Derivative2 ==
  note: U(k)
  note: ( U(k) - U(k-1) )
  U : Inport
  Data Type Duplicate : DataTypeDuplicate  DisableCoverage=on  NumInputPorts=3
  Diff : Sum  Description=Add in CPU  Inputs=+-  OutMin=OutMin  OutMax=OutMax  OutDataTypeStr=diffDT
  TSamp : SampleTimeMath  DisableCoverage=on  TsampMathOp=/  weightValue=inverseGainval  TsampMathImp=Offline Scaling Adjustment
  UD : UnitDelay  Description=Store in Global RAM  DisableCoverage=on  InitialCondition=ICPrevScaledInput  SampleTime=-1  HasFrameUpgradeWarning=on
  Y : Outport  OutMin=OutMin  OutMax=OutMax  InitialOutput=0
  wires:
  TSamp/1 -> Data Type Duplicate/2, Diff/1, UD/1
  Diff/1 -> Data Type Duplicate/1, Y/1
  UD/1 -> Data Type Duplicate/3, Diff/2  "U(k-1)"
  U/1 -> TSamp/1

== system sat_model_delivery/Control/Discrete Varying Lowpass2 ==
  u : Inport
  frequency : Inport  Port=2
  FOS : cstextras/DiscreteFirstOrderSection  VariantControl=(default)  Ts=Ts  w0=w0
  y : Outport  VectorParamsAs1DForOutWhenUnconnected=off
  wires:
  FOS/1 -> y/1
  frequency/1 -> FOS/2
  u/1 -> FOS/1

== system sat_model_delivery/Control/Slew Maneuver ==
  Abn_sens : Inport
  A_nl : Inport  Port=2
  B_m : Inport  Port=3
  Enable : EnablePort
  Control Logic : Subsystem
  Gain : Gain  Gain=-0.6
  Gain2 : Gain  Gain=-0.001
  Matrix Multiply : Product  Multiplication=Matrix(*)
  Sum : Sum
  To Workspace : ToWorkspace  VariableName=u  SampleTime=-1
  compute alphadots : Subsystem
  compute alphas : Subsystem
  cmd : Outport
  wires:
  A_nl/1 -> Matrix Multiply/2
  Abn_sens/1 -> Matrix Multiply/1, compute alphadots/1(Abn)
  Matrix Multiply/1 -> compute alphadots/2(Abl), compute alphas/1(Abl)
  compute alphadots/1(Alphadots) -> Gain/1
  compute alphas/1(estimated state) -> Gain2/1
  Gain/1 -> Sum/1
  Gain2/1 -> Sum/2
  B_m/1 -> Control Logic/2(B_m)
  Sum/1 -> Control Logic/1(u), To Workspace/1
  Control Logic/1(cmd) -> cmd/1

== system sat_model_delivery/Environment/Disturbances ==
  Abl : Inport
  R_N : Inport  Port=2
  B_b : Inport  Port=3
  flag_detumb : Inport  Port=4
  Constant : Constant  Value=[1; 0; 0]
  "Magnetic Torque " : Subsystem
  Matrix Multiply : Product  Multiplication=Matrix(*)
  Sum : Sum  Inputs=|++
  gravity torque : Subsystem
      settings: PortSchema="{\"entries\":[{\"content\":{\"sides\":[{\"content\":{\"connectorIds\":[\"In1\",\"In2\"]},\"type\":\"ConnectorPlacement.EquallySpacedRectSide\",\"uuid\":\"d49d6870-6e18-442d-ac3f-0ffb99db4fb9\"},{\"content\":{\"connectorIds\":[\"Out1\"],\"side\":\"RIGHT\"},\"type\":\"ConnectorPlacement.EquallySpacedRectSide\",\"uuid\":\"51768b95-ad39-4529-996f-06c4eddcfd5b\"},{\"content\":{\"connectorIds\":[\"In3\"],\"side\":\"TOP\"},\"type\":\"ConnectorPlacement.EquallySpacedRectSide\",\"uuid\":\"e663e83e-de9b-4162-bf16-48c6c9fc5e6f\"}]},\"type\":\"ConnectorPlacement.EquallySpacedConnector\",\"uuid\":\"e38cf75e-8247-48a0-ac18-4beb5471123c\"}],\"packageUris\":[\"http://schema.mathworks.com/mf0/Connector/R2020b\"],\"version\":\"1.0\"}"
  norm : Subsystem
  M_dist : Outport
  wires:
  Abl/1 -> Matrix Multiply/1
  Constant/1 -> Matrix Multiply/2
  Matrix Multiply/1 -> gravity torque/1(c)
  R_N/1 -> norm/1(rn)
  gravity torque/1(M_g) -> Sum/1
  "Magnetic Torque "/1(M_m) -> Sum/2
  Sum/1 -> M_dist/1
  norm/1(rnorm) -> gravity torque/2(rnorm)
  B_b/1 -> "Magnetic Torque "/1(B_b)
  flag_detumb/1 -> gravity torque/3(flag_detumb)

== system sat_model_delivery/Environment/Keplerian Dynamics ==
  A_np : Constant  Value=A_pn'
  Constant : Constant  Value=0
  Constant1 : Constant  Value=e
  Cos : Trigonometry  Operator=cos
  Integrator : Integrator
  Matrix Multiply : Product  Multiplication=Matrix(*)
  Product2 : Product
  Sin : Trigonometry
  Vector Concatenate : Concatenate  NumInputs=3
  r_norm : Subsystem
  theta integration : Subsystem
      settings: PortSchema="{\"entries\":[{\"content\":{\"sides\":[{\"content\":{\"connectorIds\":[\"In1\"]},\"type\":\"ConnectorPlacement.EquallySpacedRectSide\",\"uuid\":\"3f1b1ec9-07ed-4eb1-9e41-630dc5613e97\"},{\"content\":{\"connectorIds\":[\"Out1\",\"In2\"],\"side\":\"RIGHT\"},\"type\":\"ConnectorPlacement.EquallySpacedRectSide\",\"uuid\":\"22d0f7bc-714c-4365-a26c-07047ff4be14\"},{\"content\":{\"side\":\"TOP\"},\"type\":\"ConnectorPlacement.EquallySpacedRectSide\",\"uuid\":\"875f7006-d698-4730-93ae-1a7d05f24054\"}]},\"type\":\"ConnectorPlacement.EquallySpacedConnector\",\"uuid\":\"799b65b1-faea-432b-9f3f-2d21984184cd\"}],\"packageUris\":[\"http://schema.mathworks.com/mf0/Connector/R2020b\"],\"version\":\"1.0\"}"
  R_N : Outport
  theta : Outport  Port=2
  wires:
  Integrator/1 -> r_norm/2(theta), theta/1, Sin/1, Cos/1, theta integration/1(theta)
  theta integration/1(theta_dot) -> Integrator/1
  Constant/1 -> Vector Concatenate/3
  Cos/1 -> Vector Concatenate/1
  Constant1/1 -> theta integration/2(e), r_norm/1(e)
  r_norm/1(r) -> Product2/1
  Vector Concatenate/1 -> Product2/2
  Sin/1 -> Vector Concatenate/2
  A_np/1 -> Matrix Multiply/1
  Product2/1 -> Matrix Multiply/2
  Matrix Multiply/1 -> R_N/1

== system sat_model_delivery/Environment/Magnetic Field ==
  R_N : Inport
  Cartesian to Spherical : simulink_extras/Transformations/Cartesian to Spherical
  Constant : Constant  Value=gh
  Demux : Demux  Outputs=3
  MATLAB Function : MATLAB Function  TreatAsAtomicUnit=on
  Matrix Multiply : Product  Multiplication=Matrix(*)
  Matrix Multiply1 : Product  Multiplication=Matrix(*)
  R_en : Subsystem
  Transpose : Math  Operator=transpose
  B_N : Outport
  wires:
  R_en/1(R_en) -> Transpose/1, Matrix Multiply/1
  Demux/1 -> Cartesian to Spherical/1
  Demux/2 -> Cartesian to Spherical/2
  Demux/3 -> Cartesian to Spherical/3
  Matrix Multiply/1 -> Demux/1
  Cartesian to Spherical/1 -> MATLAB Function/1(r)
  Cartesian to Spherical/2 -> MATLAB Function/2(theta)
  Cartesian to Spherical/3 -> MATLAB Function/3(phi)
  Transpose/1 -> Matrix Multiply1/1
  MATLAB Function/1(B) -> Matrix Multiply1/2
  Constant/1 -> MATLAB Function/4(gh)
  R_N/1 -> Matrix Multiply/2
  Matrix Multiply1/1 -> B_N/1

== system sat_model_delivery/Environment/Relative Kinematics ==
  A_bn : Inport
  theta : Inport  Port=2
  Constant : Constant  Value=A_pn'
  Matrix Multiply : Product  Multiplication=Matrix(*)
  Matrix Multiply2 : Product  Multiplication=Matrix(*)
  Subsystem : Subsystem
  A_bl : Outport
  A_nl : Outport  Port=2
  wires:
  A_bn/1 -> Matrix Multiply2/1
  Matrix Multiply/1 -> A_nl/1, Matrix Multiply2/2  "A_nl"
  Matrix Multiply2/1 -> A_bl/1
  theta/1 -> Subsystem/1(theta)
  Subsystem/1(A_pl) -> Matrix Multiply/2  "A_pl"
  Constant/1 -> Matrix Multiply/1  "A_np"

== system sat_model_delivery/Environment/compute alphas ==
  Abl : Inport
  Selector6 : Selector  NumberOfDimensions=2  InputPortWidth=3  IndexOptions=Index vector (dialog),Index vector (dialog)  Indices=3,2  OutputSizes=1,1
  Selector7 : Selector  NumberOfDimensions=2  InputPortWidth=3  IndexOptions=Index vector (dialog),Index vector (dialog)  Indices=1,3  OutputSizes=1,1
  Selector8 : Selector  NumberOfDimensions=2  InputPortWidth=3  IndexOptions=Index vector (dialog),Index vector (dialog)  Indices=2,1  OutputSizes=1,1
  Sum3 : Sum  Inputs=|+-
  Transpose : Math  Operator=transpose
  Vector Concatenate1 : Concatenate  NumInputs=3
  estimated state : Outport
  wires:
  Abl/1 -> Sum3/2, Transpose/1
  Transpose/1 -> Sum3/1
  Sum3/1 -> Selector8/1, Selector7/1, Selector6/1
  Vector Concatenate1/1 -> estimated state/1
  Selector7/1 -> Vector Concatenate1/2
  Selector6/1 -> Vector Concatenate1/1
  Selector8/1 -> Vector Concatenate1/3

== system sat_model_delivery/Kinematics/Kinematics 312 ==
  w : Inport
  Enable : EnablePort  StatesWhenEnabling=reset
  A - s_312 : Subsystem
  Euler angles : Subsystem
  IC : InitialCondition  Value=s0
  s_312 - A : Subsystem
  s_313 - A : Subsystem
  A : Outport
  wires:
  s_312 - A/1(A) -> A/1  "A"
  Euler angles/1(s) -> s_312 - A/1(s)  "s"
  w/1 -> Euler angles/1(w)
  IC/1 -> Euler angles/2(s0)
  A - s_312/1(s) -> IC/1
  s_313 - A/1(A) -> A - s_312/1(A)
  [s_313] -> s_313 - A/1(s)

== system sat_model_delivery/Kinematics/Kinematics 313 ==
  w : Inport
  Enable : EnablePort  StatesWhenEnabling=reset
  A - s_313 : Subsystem
  Euler angles : Subsystem
  s_312 - A : Subsystem
  s_313 - A : Subsystem
  A : Outport
  wires:
  w/1 -> Euler angles/1(w)
  Euler angles/1(s) -> s_313 - A/1(s)
  s_313 - A/1(A) -> A/1
  A - s_313/1(s) -> Euler angles/2(s0)
  s_312 - A/1(A) -> A - s_313/1(A)
  [s_312] -> s_312 - A/1(s)

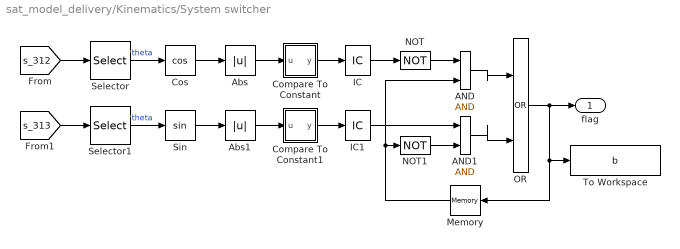
== system sat_model_delivery/Kinematics/System switcher ==
  AND : Logic  IconShape=distinctive  AllPortsSameDT=off  OutDataTypeStr=boolean
  AND1 : Logic  IconShape=distinctive  AllPortsSameDT=off  OutDataTypeStr=boolean
  Abs : Abs  SaturateOnIntegerOverflow=off
  Abs1 : Abs  SaturateOnIntegerOverflow=off
  Compare To Constant : Subsystem  mask(Compare To Constant){relop=<, const=tol, OutDataTypeStr=boolean, ZeroCross=on}
      mask prompts: relop "Simulink:masks:Operator_MP"; const "Simulink:masks:ConstantValue_MP"; OutDataTypeStr "Simulink:masks:OutputDataType_MP"; ZeroCross "Simulink:masks:EnableZerocrossingDetection_MP"
      mask help: Simulink:masks:CompareToConstant_MD
      mask init: same as sat_model_delivery/Control/De-Tumbling Bdot control1/Compare To Constant
      settings: LibrarySourceBlock=|
      | simulink/Logic and Bit
      | Operations/Compare
      | To Constant
      mask TypeOptions relop: == | ~= | < | <= | >= | >
      mask TypeOptions OutDataTypeStr: Simulink:masks:uint8 | Simulink:masks:boolean
      mask Callback ZeroCross: sl('zeroCrossEnable', gcbh);
      mask Display: disp(str)
  Compare To Constant1 : Subsystem  mask(Compare To Constant){relop=<, const=tol, OutDataTypeStr=boolean, ZeroCross=on}
      mask prompts: relop "Simulink:masks:Operator_MP"; const "Simulink:masks:ConstantValue_MP"; OutDataTypeStr "Simulink:masks:OutputDataType_MP"; ZeroCross "Simulink:masks:EnableZerocrossingDetection_MP"
      mask help: Simulink:masks:CompareToConstant_MD
      mask init: same as sat_model_delivery/Control/De-Tumbling Bdot control1/Compare To Constant
      settings: LibrarySourceBlock=|
      | simulink/Logic and Bit
      | Operations/Compare
      | To Constant
      mask TypeOptions relop: == | ~= | < | <= | >= | >
      mask TypeOptions OutDataTypeStr: Simulink:masks:uint8 | Simulink:masks:boolean
      mask Callback ZeroCross: sl('zeroCrossEnable', gcbh);
      mask Display: disp(str)
  Cos : Trigonometry  Operator=cos
  IC : InitialCondition  Value=0
  IC1 : InitialCondition  Value=0
  Memory : Memory  InitialCondition=1
  NOT : Logic  Operator=NOT  IconShape=distinctive  AllPortsSameDT=off  OutDataTypeStr=boolean
  NOT1 : Logic  Operator=NOT  IconShape=distinctive  AllPortsSameDT=off  OutDataTypeStr=boolean
  OR : Logic  Operator=OR  IconShape=distinctive  AllPortsSameDT=off  OutDataTypeStr=boolean
  Selector : Selector  InputPortWidth=3  IndexOptions=Index vector (dialog)  Indices=2  OutputSizes=1
  Selector1 : Selector  InputPortWidth=3  IndexOptions=Index vector (dialog)  Indices=2  OutputSizes=1
  Sin : Trigonometry
  To Workspace : ToWorkspace  VariableName=b  SaveFormat=Timeseries  SampleTime=-1
  flag : Outport
  wires:
  Cos/1 -> Abs/1
  [s_312] -> Selector/1
  Compare To Constant/1(y) -> IC/1
  Selector1/1 -> Sin/1  "theta"
  Abs/1 -> Compare To Constant/1(u)
  Compare To Constant1/1(y) -> IC1/1
  Selector/1 -> Cos/1  "theta"
  Abs1/1 -> Compare To Constant1/1(u)
  Sin/1 -> Abs1/1
  [s_313] -> Selector1/1
  IC/1 -> NOT/1
  NOT/1 -> AND/1
  AND/1 -> OR/1
  NOT1/1 -> AND1/2
  IC1/1 -> AND1/1
  AND1/1 -> OR/2
  OR/1 -> To Workspace/1, Memory/1, flag/1
  Memory/1 -> AND/2, NOT1/1

== system sat_model_delivery/Sensors/Earth position ==
  A_bn : Inport
  R_N : Inport  Port=2
  Matrix Multiply : Product  Multiplication=Matrix(*)
  Normalize Vector1 : vrlib/Utilities/Normalize Vector  maxzero=0
  To Workspace : ToWorkspace  VariableName=rb  SampleTime=-1
  Zero-Order Hold : ZeroOrderHold  SampleTime=1/freq_acds
  r_b : Outport
  v_h : Outport  Port=2
  wires:
  Normalize Vector1/1 -> Zero-Order Hold/1, Matrix Multiply/2
  Matrix Multiply/1 -> To Workspace/1, r_b/1
  R_N/1 -> Normalize Vector1/1
  A_bn/1 -> Matrix Multiply/1
  Zero-Order Hold/1 -> v_h/1
